simulink subsystem "Evitador_Paredes_Controlador"  (R2023b)
settings: Solver=VariableStepAuto  StartTime=0.0  StopTime=10.0  RelTol=1e-3
settings Model: Creator=juana  LastModifiedBy=juana

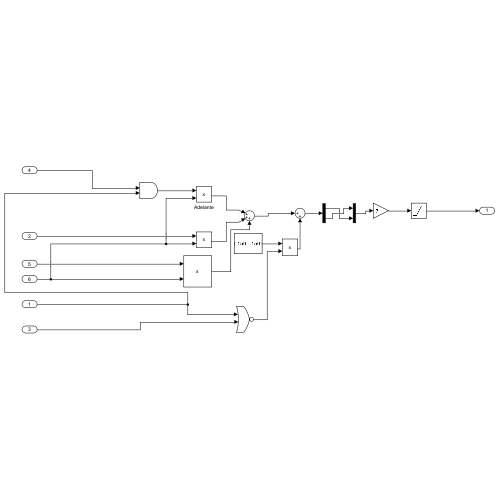
[thumbnail: Simulink's stored preview of the top-level diagram]
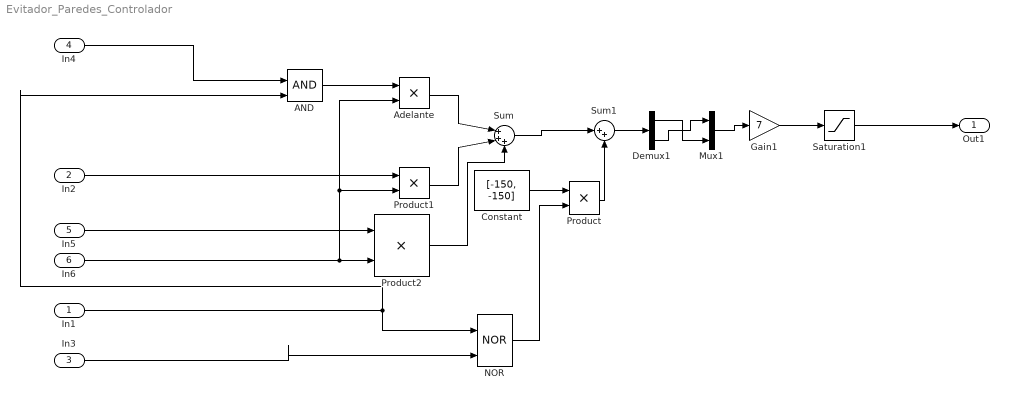
== system Evitador_Paredes_Controlador ==
  In1 : Inport
  In2 : Inport  Port=2
  In3 : Inport  Port=3
  In4 : Inport  Port=4
  In5 : Inport  Port=5
  In6 : Inport  Port=6
  AND : Logic  IconShape=distinctive  AllPortsSameDT=off  OutDataTypeStr=boolean
  Adelante : Product
  Constant : Constant  Value=[-150, -150]
  Demux1 : Demux  Outputs=2
  Gain1 : Gain  Gain=7  OutDataTypeStr=int64
  Mux1 : Mux  Inputs=2
  NOR : Logic  Operator=NOR  IconShape=distinctive  AllPortsSameDT=off  OutDataTypeStr=boolean
  Product : Product
  Product1 : Product
  Product2 : Product
  Saturation1 : Saturate  UpperLimit=180  LowerLimit=-180  OutMin=[-255]  OutMax=[255]  OutDataTypeStr=int64
  Sum : Sum  Inputs=|+++
  Sum1 : Sum  Inputs=|++
  Out1 : Outport
  wires:
  Product2/1 -> Sum/3
  Adelante/1 -> Sum/1
  NOR/1 -> Product/2
  Sum1/1 -> Demux1/1
  In1/1 -> AND/2, NOR/1
  In4/1 -> AND/1
  Product1/1 -> Sum/2
  Product/1 -> Sum1/2
  Sum/1 -> Sum1/1
  In6/1 -> Product2/2, Adelante/2, Product1/2
  In2/1 -> Product1/1
  AND/1 -> Adelante/1
  Demux1/1 -> Mux1/2
  In5/1 -> Product2/1
  Mux1/1 -> Gain1/1
  In3/1 -> NOR/2
  Gain1/1 -> Saturation1/1
  Constant/1 -> Product/1
  Demux1/2 -> Mux1/1
  Saturation1/1 -> Out1/1
